simulink model "enabled"  (R2018a)
settings: Solver=ode45  StartTime=0.0  StopTime=10.0  RelTol=1e-3  EnableMultiTasking=on
libraries: simulink x1
settings Model: Creator=nicholas  LastModifiedBy=bneiswan
settings DataIOCC: LimitDataPoints=on  SaveFormat=Array  SignalLoggingName=sigsOut
settings OptimizationCC: ExpressionDepthLimit=2147483647  InitFltsAndDblsToZero=on  LifeSpan=inf
settings DebuggingCC: SaveWithParameterizedLinksMsg=none  UnderspecifiedInitializationDetection=Classic  MergeDetectMultiDrivingBlocksExec=none  CheckExecutionContextPreStartOutputMsg=on  CheckExecutionContextRuntimeOutputMsg=on  SignalResolutionControl=TryResolveAllWithWarning  MultiTaskDSMMsg=warning  MultiTaskCondExecSysMsg=none  ParameterPrecisionLossMsg=none  FcnCallInpInsideContextMsg=warning  AllowSymbolicDim=off  StateNameClashWarn=warning  SFUnexpectedBacktrackingDiag=warning  SFNoUnconditionalDefaultTransitionDiag=warning  SFExecutionAtInitializationDiag=none
settings HardwareCC: ProdBitPerPointer=32  ProdBitPerSizeT=32  ProdBitPerPtrDiffT=32  ProdLargestAtomicFloat=None  ProdIntDivRoundTo=Undefined  ProdEndianess=Unspecified  ProdWordSize=32  ProdHWDeviceType=32-bit Generic  TargetUnknown=on
settings ModelReferenceCC: PropagateSignalLabelsOutOfModel=off
settings CodeAppCC: StateflowObjectComments=on
settings GRTTargetCC: TargetFcnLib=ansi_tfl_tmw.mat  TargetLangStandard=C89/C90 (ANSI)  GeneratePreprocessorConditionals=Disable all  CombineOutputUpdateFcns=off  GRTInterface=on
settings ConfigComp: CovMetricSettings=dw  CovHtmlReporting=on  CovSaveCumulativeToWorkspaceVar=on  CovSaveSingleToWorkspaceVar=on  CovExternalEMLEnable=off  CovSFcnEnable=off

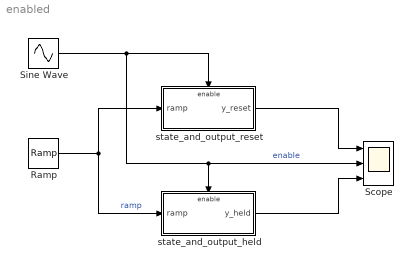
== system enabled ==
  Ramp : simulink/Sources/Ramp  slope=1  start=0  InitialOutput=0
  Scope : Scope  NumInputPorts=3
  Sine Wave : Sin  SampleTime=0
  state_and_output_held : Subsystem  TreatAsAtomicUnit=on
  state_and_output_reset : Subsystem  TreatAsAtomicUnit=on
  wires:
  Ramp/1 -> state_and_output_held/1(ramp), state_and_output_reset/1(ramp)  "ramp"
  state_and_output_held/1(y_held) -> Scope/3
  state_and_output_reset/1(y_reset) -> Scope/1
  Sine Wave/1 -> state_and_output_held/Enable, Scope/2, state_and_output_reset/Enable  "enable"

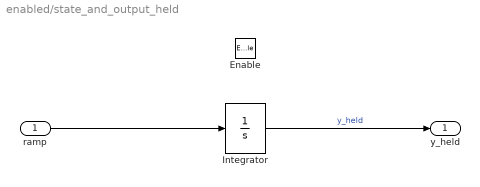
== system enabled/state_and_output_held ==
  ramp : Inport
  Enable : EnablePort
      settings: AttributesFormatString=States when enabling: %<StatesWhenEnabling>
  Integrator : Integrator
  y_held : Outport  InitialOutput=0
      settings: AttributesFormatString="Output when\\ndisabled:  %<OutputWhenDisabled>"
  wires:
  ramp/1 -> Integrator/1
  Integrator/1 -> y_held/1  "y_held"

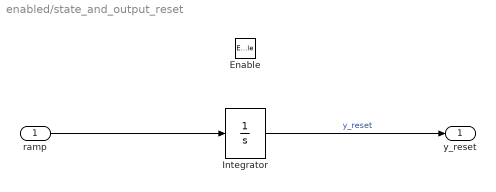
== system enabled/state_and_output_reset ==
  ramp : Inport
  Enable : EnablePort  StatesWhenEnabling=reset
      settings: AttributesFormatString=States when enabling: %<StatesWhenEnabling>
  Integrator : Integrator
  y_reset : Outport  OutputWhenDisabled=reset  InitialOutput=0
      settings: AttributesFormatString="Output when\\ndisabled:  %<OutputWhenDisabled>"
  wires:
  Integrator/1 -> y_reset/1  "y_reset"
  ramp/1 -> Integrator/1
